simulink model "PI_controller"  (R2019b)
settings: Solver=FixedStepAuto  StartTime=0.0  StopTime=5  FixedStep=0.005  RelTol=1e-3
values from neighbouring files (symbols this model uses):
  Ki = 0.3    [sim_zn1.m]
  Kp = 0.4    [sim_zn1.m]
undefined symbols (not defined in the file or in its folder): a, b
settings Model: Creator=suvo  LastModifiedBy=suvo

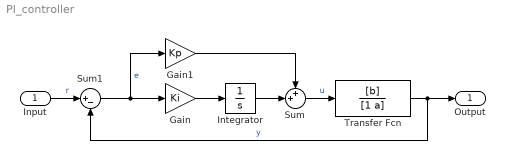
== system PI_controller ==
  Input : Inport
  Gain : Gain  Gain=Ki
  Gain1 : Gain  Gain=Kp
  Integrator : Integrator
  Sum : Sum  Inputs=++|
  Sum1 : Sum  Inputs=|+-
  Transfer Fcn : TransferFcn  Numerator=[b]  Denominator=[1 a]
  Output : Outport
  wires:
  Sum1/1 -> Gain1/1, Gain/1  "e"
  Input/1 -> Sum1/1  "r"
  Transfer Fcn/1 -> Output/1, Sum1/2  "y"
  Integrator/1 -> Sum/2
  Gain/1 -> Integrator/1
  Gain1/1 -> Sum/1
  Sum/1 -> Transfer Fcn/1  "u"
